simulink model "loop_A_s"  (R2020b)
settings: Solver=VariableStepAuto  StartTime=0.0  StopTime=10.0  RelTol=1e-3
undefined symbols (not defined in the file): Z_3, Z_345, Z_4, Z_5
libraries: cstblocks x4
settings Model: Creator=jasper  LastModifiedBy=jasper

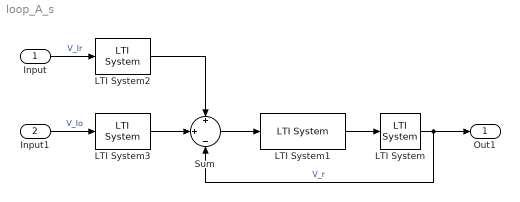
== system loop_A_s ==
  Input : Inport
  Input1 : Inport  Port=2
  LTI System : cstblocks/LTI System  sys=A_s  IC=[]
  LTI System1 : cstblocks/LTI System  sys=1/(Z_4*Z_345)  IC=[]
  LTI System2 : cstblocks/LTI System  sys=-Z_4/Z_3  IC=[]
  LTI System3 : cstblocks/LTI System  sys=-Z_4/Z_5  IC=[]
  Sum : Sum  Inputs=+|+|-
  Out1 : Outport
  wires:
  LTI System1/1 -> LTI System/1
  Sum/1 -> LTI System1/1
  LTI System/1 -> Out1/1, Sum/3  "V_r"
  LTI System3/1 -> Sum/2
  LTI System2/1 -> Sum/1
  Input/1 -> LTI System2/1  "V_Ir"
  Input1/1 -> LTI System3/1  "V_Io"
